simulink model "Motor_SimScape"  (R2021a)
settings: Solver=FixedStepAuto  StartTime=0.0  StopTime=t_end  FixedStep=dt  RelTol=1e-3
values from neighbouring files (symbols this model uses):
  Amp = 1.1    [main.m]
  angle_ini = 2*pi*id/100    [main.m]
  displacement = [desp_x;desp_y]    [main.m]
  dt = t(2)    [main.m]    (also in simulation.m = 0.001)
  g = plot(time,T_ref,time,torque)    [simulation.m]
  home = [x_home;y_home]    [main.m]
  K = 0.4    [main.m]
  K_sensor = 15    [simulation.m]
  Kd1 = 0    [simulation.m]
  Kd2 = 0    [simulation.m]
  Ki2 = 0    [simulation.m]
  Kp1 = 3.09 , Ki1 = 0    [simulation.m]
  Kp2 = 2.34    [simulation.m]
  L1 = 22    [main.m]
  L2 = 20    [main.m]
  mode = 2    [simulation.m]
  N = 1    [main.m]
  phi = -3*pi/4    (= -2.35619449019)    [main.m]
  sampling = 50    [simulation.m]
  T = 20    [main.m]
undefined symbols (not defined in the file or in its folder): b1, b2, Ki1, Ra1, Ra2, X, Y, Z
libraries: fl_lib x24, sm_lib x20, nesl_utility x17, ee_lib x6, pid_lib x2, simulink x1
(part 2 of 2)

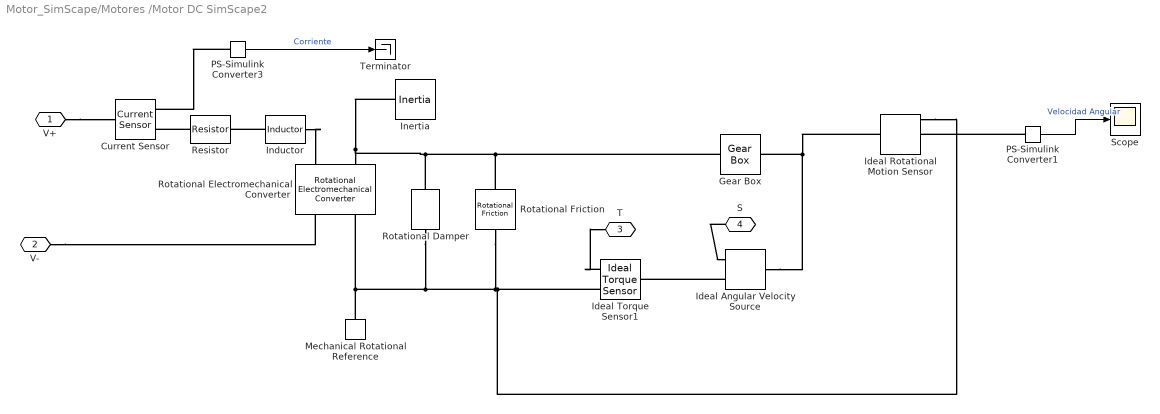
== system Motor_SimScape/Motores /Motor DC SimScape2 ==
  Current Sensor : fl_lib/Electrical/Electrical Sensors/Current Sensor
  Gear Box : fl_lib/Mechanical/Mechanisms/Gear Box  ratio=N2  t_in_specify=off  t_in_priority=None  t_in=0 N*m  t_in_nominal_specify=off  t_in_nominal_unit=N*m  t_in_nominal_value=1  t_out_specify=off  t_out_priority=None  t_out=0 N*m  t_out_nominal_specify=off  t_out_nominal_unit=N*m  t_out_nominal_value=1
  Ideal Angular Velocity Source : fl_lib/Mechanical/Mechanical Sources/Ideal Angular Velocity Source
  Ideal Rotational Motion Sensor : fl_lib/Mechanical/Mechanical Sensors/Ideal Rotational Motion Sensor  wrap_angle=simscape.enum.onoff.off  offset=0 rad
  Ideal Torque Sensor1 : fl_lib/Mechanical/Mechanical Sensors/Ideal Torque Sensor
  Inductor : ee_lib/Passive/Inductor  l=La2 H  L_tol=20  enable_L_tol=0  tol_distribution=1  nSigma=4  r=0 Ohm  g=1e-9 1/Ohm  enable_operating_limits=0  operating_limit_action=2  max_working_current=1 A  power_rating=1 W  enable_faults=0  fault_action=1  lambdaPercent=50  k_faulted=0.9999  turnsShort=0  openCct=0  groundShort=0  groundShortG=0 1/Ohm  tau_fault=1e-3 s  enable_temporal_fault=0  t_fault=1 s  enable_behavioral_fault=0  max_permissible_voltage=100 V  n_fail_on_voltage=1  max_permissible_current=1 A  t_fail_on_current=1 s  i_L_specify=off  i_L_priority=High  i_L=0 A  i_L_nominal_specify=off  i_L_nominal_unit=A  i_L_nominal_value=1
  Inertia : fl_lib/Mechanical/Rotational Elements/Inertia  inertia=JM2 kg*m^2  num_ports=foundation.enum.numPorts2.one  w_specify=off  w_priority=High  w=0 rad/s  w_nominal_specify=off  w_nominal_unit=rad/s  w_nominal_value=1  t_specify=off  t_priority=None  t=0 N*m  t_nominal_specify=off  t_nominal_unit=N*m  t_nominal_value=1
  Mechanical Rotational Reference : fl_lib/Mechanical/Rotational Elements/Mechanical Rotational Reference
  PS-Simulink Converter1 : nesl_utility/PS-Simulink Converter  PhysicalDomain=network_engine_domain  SubClassName=ps_output  LeftPortType=input  RightPortType=output  PseudoPeriodic=off  Frequencies=[]  Unit=rad/s  AffineConversion=off
      settings: SourceProductBaseCode=PW,SS
  PS-Simulink Converter3 : nesl_utility/PS-Simulink Converter  PhysicalDomain=network_engine_domain  SubClassName=ps_output  LeftPortType=input  RightPortType=output  PseudoPeriodic=off  Frequencies=[]  Unit=inherit  AffineConversion=off
      settings: SourceProductBaseCode=PW,SS
  Resistor : ee_lib/Passive/Resistor  R=Ra2 Ohm  R_tol=5  enable_R_tol=0  tol_distribution=1  nSigma=4  enable_operating_limits=0  operating_limit_action=2  max_working_voltage=100 V  power_rating=1 W  enable_faults=0  fault_action=1  R_faulted=inf Ohm  enable_temporal_fault=0  t_fault=1 s  enable_behavioral_fault=0  max_permissible_current=1 A  t_fail_on_current=1 s  noise_mode=0  sample_time=1e-3 s  repeatability=1  auto_seed=1847726676  user_seed=0  Tdevice=25 degC  alpha=3.93e-3 1/K  Tmeas=25 degC  thermal_mass=100 J/K  power_derating_T1=70 degC  power_derating_T2=155 degC  operating_temperature_range_vec=[-50, 150] degC  temperature_specify=off  temperature_priority=High  temperature=298.15 K  temperature_nominal_specify=off  temperature_nominal_unit=K  temperature_nominal_value=1
  Rotational Electromechanical Converter : fl_lib/Electrical/Electrical Elements/Rotational Electromechanical Converter  K=0.0145 V/(rad/s)  i_specify=off  i_priority=None  i=0 A  i_nominal_specify=off  i_nominal_unit=A  i_nominal_value=1  v_specify=off  v_priority=None  v=0 V  v_nominal_specify=off  v_nominal_unit=V  v_nominal_value=1  t_specify=off  t_priority=None  t=0 N*m  t_nominal_specify=off  t_nominal_unit=N*m  t_nominal_value=1  w_specify=off  w_priority=None  w=0 rad/s  w_nominal_specify=off  w_nominal_unit=rad/s  w_nominal_value=1
  Rotational Damper : fl_lib/Mechanical/Rotational Elements/Rotational Damper  D=b2 N*m/(rad/s)  w_specify=off  w_priority=None  w=0 rad/s  w_nominal_specify=off  w_nominal_unit=rad/s  w_nominal_value=1  t_specify=off  t_priority=None  t=0 N*m  t_nominal_specify=off  t_nominal_unit=N*m  t_nominal_value=1
  Rotational Friction : fl_lib/Mechanical/Rotational Elements/Rotational Friction  brkwy_trq=2e-2 N*m  brkwy_vel=1.6522e-06 rad/s  Col_trq=2e-2 N*m  visc_coef=0.02 N*m/(rad/s)  w_specify=off  w_priority=None  w=0 rad/s  w_nominal_specify=off  w_nominal_unit=rad/s  w_nominal_value=1  t_specify=off  t_priority=None  t=0 N*m  t_nominal_specify=off  t_nominal_unit=N*m  t_nominal_value=1
  Scope : Scope
  Terminator : Terminator
  V+ : PMIOPort  Side=Left
  V- : PMIOPort  Port=2  Side=Left
  T : PMIOPort  Port=3  Side=Right
  S : PMIOPort  Port=4  Side=Right
  wires:
  PS-Simulink Converter3/1 -> Terminator/1  "Corriente"
  PS-Simulink Converter1/1 -> Scope/1  "Velocidad Angular"
  connections:
  Rotational Damper/LConn1 -- Ideal Rotational Motion Sensor/RConn1 -- Ideal Torque Sensor1/RConn1 -- Rotational Friction/RConn1 -- Mechanical Rotational Reference/LConn1 -- Rotational Electromechanical Converter/RConn2
  Inductor/RConn1 -- Rotational Electromechanical Converter/LConn1
  V-/RConn1 -- Rotational Electromechanical Converter/RConn1
  Inductor/LConn1 -- Resistor/RConn1
  Resistor/LConn1 -- Current Sensor/RConn2
  V+/RConn1 -- Current Sensor/LConn1
  PS-Simulink Converter3/LConn1 -- Current Sensor/RConn1
  Inertia/LConn1 -- Gear Box/LConn1 -- Rotational Friction/LConn1 -- Rotational Damper/RConn1 -- Rotational Electromechanical Converter/LConn2
  Ideal Torque Sensor1/RConn2 -- T/RConn1
  PS-Simulink Converter1/LConn1 -- Ideal Rotational Motion Sensor/RConn2
  Ideal Angular Velocity Source/RConn2 -- Ideal Torque Sensor1/LConn1
  S/RConn1 -- Ideal Angular Velocity Source/RConn1
  Ideal Angular Velocity Source/LConn1 -- Gear Box/RConn1 -- Ideal Rotational Motion Sensor/LConn1

== matlab function Motor_SimScape/Subsystem/inverse_kinematic ==
  data: t input; T input; L1 input; L2 input; displacement input; home input; theta1 output; theta2 output; angle_ini input; Amp input; phi input; K input
function [theta1,theta2]=inverse_kinematic(t,T,L1,L2, displacement,home,angle_ini,Amp,phi,K) 

% Distancia [cm]
desp_x=displacement(1);
desp_y=displacement(2);

x_home=home(1); 
y_home=home(2);

% Parametros de trayectoria trevol estilizado

angle=2*pi*t/T+angle_ini;

r_base=8.5;       % radio base [cm]
Amp=1.1;            % factor de escala entre 1 y 1.2
phi=-3*pi/4;       % desface
K=0.4;            % factor de estilizado entre 0 y 1  
r_max=Amp*r_base*(1+K);

r=Amp*r_base*(1-K*cos(4*angle-phi));


% Desplazamiento de trayectoria
[x,y]=pol2cart(angle,r);  

x=x+desp_x;
y=y+desp_y;

d=sqrt((x-x_home).^2+(y-y_home).^2);
vel=r_max*2*pi/T;

t_start=d/vel;


if(t<t_start)  
  x=x_home+(x-x_home)*t/t_start;
  y=y_home+(y-y_home)*t/t_start;
else

end

[angle,r]=cart2pol(x,y);
L=sqrt(x.^2+y.^2);

% perfil de movimiento
theta=[angle-acos((L.^2+L1^2-L2^2)./(2*L*L1));
             acos((L.^2-L1^2-L2^2)/(2*L1*L2))];
theta1=theta(1);
theta2=theta(2);

end
